simulink model "testOpenLoop"  (R2021a)
settings: Solver=VariableStepAuto  StartTime=0.0  StopTime=Torb  RelTol=1e-3
values from neighbouring files (symbols this model uses):
  t0x = tfy + 10    [control_1.m]    (also in control_extra2.m)
  t0y = tfz + 10    [control_1.m]    (also in control_extra2.m)
  t0z = 10    [control_1.m]    (also in control_2.m; control_extra2.m)
  t_thrust = 1    [control_1.m]    (also in control_2.m; control_3.m; control_4.m; control_extra2.m)
  tfx = t0x + tx    [control_1.m]    (also in control_extra2.m)
  tfy = t0y + ty    [control_1.m]    (also in control_extra2.m)
  tfz = t0z + tz    [control_1.m]    (also in control_2.m; control_extra2.m)
  Tmax = Fmax*Larm    (= 0.00125)    [control_1.m]    (also in control_2.m; control_extra2.m)
libraries: sharedtransform x1
settings Model: DataDictionary=databus.sldd  Creator=Laura  LastModifiedBy=Laura

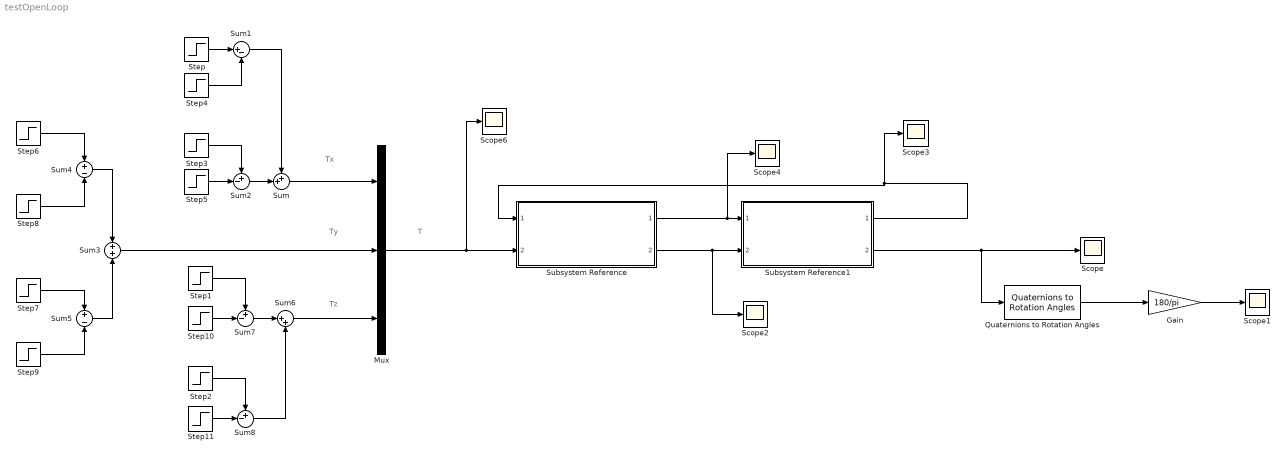
== system testOpenLoop ==
  note: Tx
  note: Ty
  note: Tz
  note: T
  Gain : Gain  Gain=180/pi
  Mux : Mux  Inputs=3
  Quaternions to Rotation Angles : sharedtransform/Quaternions to Rotation Angles  rotationOrder=ZYX  aMode=aMode
      settings: SourceProductBaseCode=AE,PW,DR,MT,UV,VE
  Scope{,1..4,6} (6 alike) : Scope
  Step : Step  Time=t0x  After=Tmax  SampleTime=0
  Step1 : Step  Time=t0z  After=Tmax  SampleTime=0
  Step10 : Step  Time=t0z + t_thrust  After=Tmax  SampleTime=0
  Step11 : Step  Time=tfz + t_thrust  After=-Tmax  SampleTime=0
  Step2 : Step  Time=tfz  After=-Tmax  SampleTime=0
  Step3 : Step  Time=tfx  After=-Tmax  SampleTime=0
  Step4 : Step  Time=t0x + t_thrust  After=Tmax  SampleTime=0
  Step5 : Step  Time=tfx + t_thrust  After=-Tmax  SampleTime=0
  Step6 : Step  Time=t0y  After=Tmax  SampleTime=0
  Step7 : Step  Time=tfy  After=-Tmax  SampleTime=0
  Step8 : Step  Time=t0y + t_thrust  After=Tmax  SampleTime=0
  Step9 : Step  Time=tfy + t_thrust  After=-Tmax  SampleTime=0
  Subsystem Reference : Subsystem  ReferencedSubsystem=Dynamics
  Subsystem Reference1 : Subsystem  ReferencedSubsystem=Kinematics
  Sum : Sum  Inputs=++|
  Sum1 : Sum  Inputs=|+-
  Sum2 : Sum  Inputs=+-|
  Sum3 : Sum
  Sum4 : Sum  Inputs=+-
  Sum5 : Sum  Inputs=+-
  Sum6 : Sum  Inputs=|++
  Sum7 : Sum  Inputs=+-|
  Sum8 : Sum  Inputs=+-|
  wires:
  Subsystem Reference1/1 -> Scope3/1, Subsystem Reference/1
  Subsystem Reference1/2 -> Quaternions to Rotation Angles/1, Scope/1
  Subsystem Reference/2 -> Scope2/1, Subsystem Reference1/2
  Subsystem Reference/1 -> Scope4/1, Subsystem Reference1/1
  Step/1 -> Sum1/1
  Sum1/1 -> Sum/1
  Step4/1 -> Sum1/2
  Sum/1 -> Mux/1
  Step3/1 -> Sum2/1
  Step5/1 -> Sum2/2
  Sum2/1 -> Sum/2
  Sum4/1 -> Sum3/1
  Step6/1 -> Sum4/1
  Step8/1 -> Sum4/2
  Sum5/1 -> Sum3/2
  Step7/1 -> Sum5/1
  Step9/1 -> Sum5/2
  Sum3/1 -> Mux/2
  Sum8/1 -> Sum6/2
  Step10/1 -> Sum7/2
  Step11/1 -> Sum8/2
  Step1/1 -> Sum7/1
  Sum7/1 -> Sum6/1
  Step2/1 -> Sum8/1
  Sum6/1 -> Mux/3
  Mux/1 -> Scope6/1, Subsystem Reference/2
  Quaternions to Rotation Angles/1 -> Gain/1
  Gain/1 -> Scope1/1
